simulink model "GalacticSoupLogical"  (R2026a)
settings: Solver=VariableStepAuto
settings Model: DataDictionary=LogicalInterfaces.sldd  Creator=sarah  LastModifiedBy=sarah

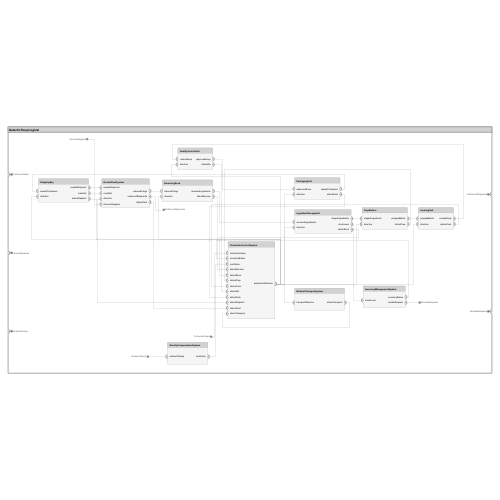
[thumbnail: Simulink's stored preview of the top-level diagram]
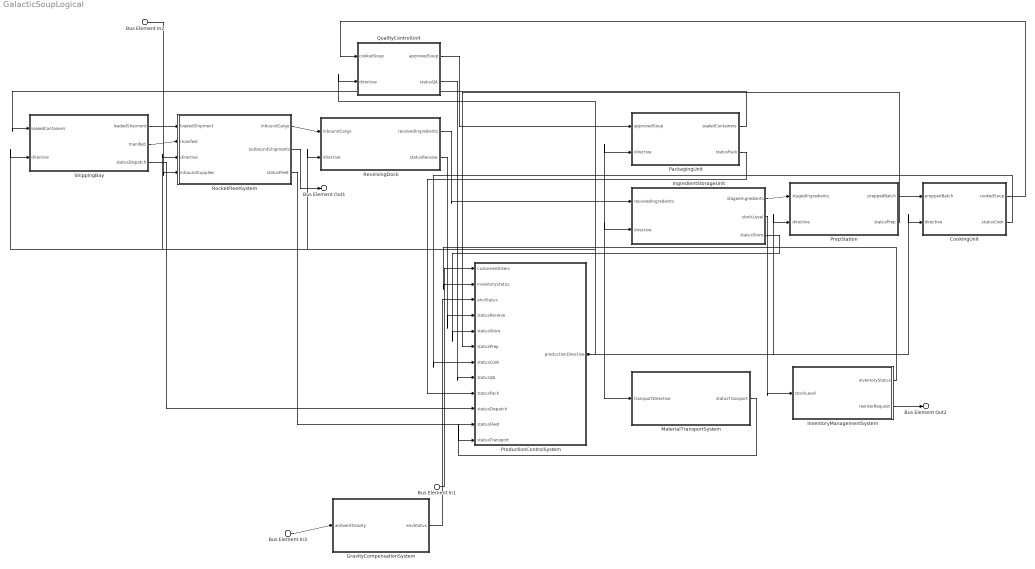
== system GalacticSoupLogical ==
  Bus Element In1 : Inport  PortName=CustomerOrders
  Bus Element In2 : Inport  Port=2  PortName=InboundSupplies
  Bus Element In3 : Inport  Port=3  PortName=AmbientGravity
  CookingUnit : Subsystem
      settings: PortSchema="{\"entries\":[{\"content\":{\"headerSize\":26,\"margin\":15,\"minimumSpacing\":25,\"sides\":[{\"content\":{\"connectorIds\":[\"In1\",\"In2\"]},\"type\":\"ConnectorPlacement.EquallySpacedRectSide\",\"uuid\":\"f830f98a-8e8b-4468-adf4-d6eab644987f\"},{\"content\":{\"connectorIds\":[\"Out1\",\"Out2\"],\"side\":\"RIGHT\"},\"type\":\"ConnectorPlacement.EquallySpacedRectSide\",\"uuid\":\"7e0d0116-b3ba-4668-b638-30d0f54ba087\"},{\"content\":{\"side\":\"TOP\"},\"type\":\"ConnectorPlacement.EquallySpacedRectSide\",\"uuid\":\"7b4146d3-46d2-45ca-8c34-b106f0d8cedd\"}]},\"type\":\"ConnectorPlacement.EquallySpacedConnector\",\"uuid\":\"3d911b2d-a78f-42ea-b869-5e09982d9f54\"}],\"packageUris\":[\"http://schema.mathworks.com/mf0/Connector/R2020b\"],\"version\":\"1.0\"}"
  GravityCompensationSystem : Subsystem
      settings: PortSchema="{\"entries\":[{\"content\":{\"headerSize\":26,\"margin\":15,\"minimumSpacing\":25,\"sides\":[{\"content\":{\"connectorIds\":[\"In1\"]},\"type\":\"ConnectorPlacement.EquallySpacedRectSide\",\"uuid\":\"f830f98a-8e8b-4468-adf4-d6eab644987f\"},{\"content\":{\"connectorIds\":[\"Out1\"],\"side\":\"RIGHT\"},\"type\":\"ConnectorPlacement.EquallySpacedRectSide\",\"uuid\":\"7e0d0116-b3ba-4668-b638-30d0f54ba087\"},{\"content\":{\"side\":\"TOP\"},\"type\":\"ConnectorPlacement.EquallySpacedRectSide\",\"uuid\":\"7b4146d3-46d2-45ca-8c34-b106f0d8cedd\"}]},\"type\":\"ConnectorPlacement.EquallySpacedConnector\",\"uuid\":\"3d911b2d-a78f-42ea-b869-5e09982d9f54\"}],\"packageUris\":[\"http://schema.mathworks.com/mf0/Connector/R2020b\"],\"version\":\"1.0\"}"
  IngredientStorageUnit : Subsystem
      settings: PortSchema="{\"entries\":[{\"content\":{\"headerSize\":26,\"margin\":15,\"minimumSpacing\":25,\"sides\":[{\"content\":{\"connectorIds\":[\"In1\",\"In2\"]},\"type\":\"ConnectorPlacement.EquallySpacedRectSide\",\"uuid\":\"f830f98a-8e8b-4468-adf4-d6eab644987f\"},{\"content\":{\"connectorIds\":[\"Out1\",\"Out2\",\"Out3\"],\"side\":\"RIGHT\"},\"type\":\"ConnectorPlacement.EquallySpacedRectSide\",\"uuid\":\"7e0d0116-b3ba-4668-b638-30d0f54ba087\"},{\"content\":{\"side\":\"TOP\"},\"type\":\"ConnectorPlacement.EquallySpacedRectSide\",\"uuid\":\"7b4146d3-46d2-45ca-8c34-b106f0d8cedd\"}]},\"type\":\"ConnectorPlacement.EquallySpacedConnector\",\"uuid\":\"3d911b2d-a78f-42ea-b869-5e09982d9f54\"}],\"packageUris\":[\"http://schema.mathworks.com/mf0/Connector/R2020b\"],\"version\":\"1.0\"}"
  InventoryManagementSystem : Subsystem
      settings: PortSchema="{\"entries\":[{\"content\":{\"headerSize\":26,\"margin\":15,\"minimumSpacing\":25,\"sides\":[{\"content\":{\"connectorIds\":[\"In1\"]},\"type\":\"ConnectorPlacement.EquallySpacedRectSide\",\"uuid\":\"f830f98a-8e8b-4468-adf4-d6eab644987f\"},{\"content\":{\"connectorIds\":[\"Out1\",\"Out2\"],\"side\":\"RIGHT\"},\"type\":\"ConnectorPlacement.EquallySpacedRectSide\",\"uuid\":\"7e0d0116-b3ba-4668-b638-30d0f54ba087\"},{\"content\":{\"side\":\"TOP\"},\"type\":\"ConnectorPlacement.EquallySpacedRectSide\",\"uuid\":\"7b4146d3-46d2-45ca-8c34-b106f0d8cedd\"}]},\"type\":\"ConnectorPlacement.EquallySpacedConnector\",\"uuid\":\"3d911b2d-a78f-42ea-b869-5e09982d9f54\"}],\"packageUris\":[\"http://schema.mathworks.com/mf0/Connector/R2020b\"],\"version\":\"1.0\"}"
  MaterialTransportSystem : Subsystem
      settings: PortSchema="{\"entries\":[{\"content\":{\"headerSize\":26,\"margin\":15,\"minimumSpacing\":25,\"sides\":[{\"content\":{\"connectorIds\":[\"In1\"]},\"type\":\"ConnectorPlacement.EquallySpacedRectSide\",\"uuid\":\"f830f98a-8e8b-4468-adf4-d6eab644987f\"},{\"content\":{\"connectorIds\":[\"Out1\"],\"side\":\"RIGHT\"},\"type\":\"ConnectorPlacement.EquallySpacedRectSide\",\"uuid\":\"7e0d0116-b3ba-4668-b638-30d0f54ba087\"},{\"content\":{\"side\":\"TOP\"},\"type\":\"ConnectorPlacement.EquallySpacedRectSide\",\"uuid\":\"7b4146d3-46d2-45ca-8c34-b106f0d8cedd\"}]},\"type\":\"ConnectorPlacement.EquallySpacedConnector\",\"uuid\":\"3d911b2d-a78f-42ea-b869-5e09982d9f54\"}],\"packageUris\":[\"http://schema.mathworks.com/mf0/Connector/R2020b\"],\"version\":\"1.0\"}"
  PackagingUnit : Subsystem
      settings: PortSchema="{\"entries\":[{\"content\":{\"headerSize\":26,\"margin\":15,\"minimumSpacing\":25,\"sides\":[{\"content\":{\"connectorIds\":[\"In1\",\"In2\"]},\"type\":\"ConnectorPlacement.EquallySpacedRectSide\",\"uuid\":\"f830f98a-8e8b-4468-adf4-d6eab644987f\"},{\"content\":{\"connectorIds\":[\"Out1\",\"Out2\"],\"side\":\"RIGHT\"},\"type\":\"ConnectorPlacement.EquallySpacedRectSide\",\"uuid\":\"7e0d0116-b3ba-4668-b638-30d0f54ba087\"},{\"content\":{\"side\":\"TOP\"},\"type\":\"ConnectorPlacement.EquallySpacedRectSide\",\"uuid\":\"7b4146d3-46d2-45ca-8c34-b106f0d8cedd\"}]},\"type\":\"ConnectorPlacement.EquallySpacedConnector\",\"uuid\":\"3d911b2d-a78f-42ea-b869-5e09982d9f54\"}],\"packageUris\":[\"http://schema.mathworks.com/mf0/Connector/R2020b\"],\"version\":\"1.0\"}"
  PrepStation : Subsystem
      settings: PortSchema="{\"entries\":[{\"content\":{\"headerSize\":26,\"margin\":15,\"minimumSpacing\":25,\"sides\":[{\"content\":{\"connectorIds\":[\"In1\",\"In2\"]},\"type\":\"ConnectorPlacement.EquallySpacedRectSide\",\"uuid\":\"f830f98a-8e8b-4468-adf4-d6eab644987f\"},{\"content\":{\"connectorIds\":[\"Out1\",\"Out2\"],\"side\":\"RIGHT\"},\"type\":\"ConnectorPlacement.EquallySpacedRectSide\",\"uuid\":\"7e0d0116-b3ba-4668-b638-30d0f54ba087\"},{\"content\":{\"side\":\"TOP\"},\"type\":\"ConnectorPlacement.EquallySpacedRectSide\",\"uuid\":\"7b4146d3-46d2-45ca-8c34-b106f0d8cedd\"}]},\"type\":\"ConnectorPlacement.EquallySpacedConnector\",\"uuid\":\"3d911b2d-a78f-42ea-b869-5e09982d9f54\"}],\"packageUris\":[\"http://schema.mathworks.com/mf0/Connector/R2020b\"],\"version\":\"1.0\"}"
  ProductionControlSystem : Subsystem
      settings: PortSchema="{\"entries\":[{\"content\":{\"headerSize\":26,\"margin\":15,\"minimumSpacing\":25,\"sides\":[{\"content\":{\"connectorIds\":[\"In1\",\"In2\",\"In3\",\"In4\",\"In5\",\"In6\",\"In7\",\"In8\",\"In9\",\"In10\",\"In11\",\"In12\"]},\"type\":\"ConnectorPlacement.EquallySpacedRectSide\",\"uuid\":\"f830f98a-8e8b-4468-adf4-d6eab644987f\"},{\"content\":{\"connectorIds\":[\"Out1\"],\"side\":\"RIGHT\"},\"type\":\"ConnectorPlacement.EquallySpacedRectSide\",\"uuid\":\"7e0d0116-b3ba-4668-b638-30d0f54ba087\"},{\"content\":{\"side\":\"TOP\"},\"type\":\"ConnectorPlacement.EquallySpacedRectSide\",\"uuid\":\"7b4146d3-46d2-45ca-8c34-b106f0d8cedd\"}]},\"type\":\"ConnectorPlacement.EquallySpacedConnector\",\"uuid\":\"3d911b2d-a78f-42ea-b869-5e09982d9f54\"}],\"packageUris\":[\"http://schema.mathworks.com/mf0/Connector/R2020b\"],\"version\":\"1.0\"}"
  QualityControlUnit : Subsystem
      settings: PortSchema="{\"entries\":[{\"content\":{\"headerSize\":26,\"margin\":15,\"minimumSpacing\":25,\"sides\":[{\"content\":{\"connectorIds\":[\"In1\",\"In2\"]},\"type\":\"ConnectorPlacement.EquallySpacedRectSide\",\"uuid\":\"f830f98a-8e8b-4468-adf4-d6eab644987f\"},{\"content\":{\"connectorIds\":[\"Out1\",\"Out2\"],\"side\":\"RIGHT\"},\"type\":\"ConnectorPlacement.EquallySpacedRectSide\",\"uuid\":\"7e0d0116-b3ba-4668-b638-30d0f54ba087\"},{\"content\":{\"side\":\"TOP\"},\"type\":\"ConnectorPlacement.EquallySpacedRectSide\",\"uuid\":\"7b4146d3-46d2-45ca-8c34-b106f0d8cedd\"}]},\"type\":\"ConnectorPlacement.EquallySpacedConnector\",\"uuid\":\"3d911b2d-a78f-42ea-b869-5e09982d9f54\"}],\"packageUris\":[\"http://schema.mathworks.com/mf0/Connector/R2020b\"],\"version\":\"1.0\"}"
  ReceivingDock : Subsystem
      settings: PortSchema="{\"entries\":[{\"content\":{\"headerSize\":26,\"margin\":15,\"minimumSpacing\":25,\"sides\":[{\"content\":{\"connectorIds\":[\"In1\",\"In2\"]},\"type\":\"ConnectorPlacement.EquallySpacedRectSide\",\"uuid\":\"f830f98a-8e8b-4468-adf4-d6eab644987f\"},{\"content\":{\"connectorIds\":[\"Out1\",\"Out2\"],\"side\":\"RIGHT\"},\"type\":\"ConnectorPlacement.EquallySpacedRectSide\",\"uuid\":\"7e0d0116-b3ba-4668-b638-30d0f54ba087\"},{\"content\":{\"side\":\"TOP\"},\"type\":\"ConnectorPlacement.EquallySpacedRectSide\",\"uuid\":\"7b4146d3-46d2-45ca-8c34-b106f0d8cedd\"}]},\"type\":\"ConnectorPlacement.EquallySpacedConnector\",\"uuid\":\"3d911b2d-a78f-42ea-b869-5e09982d9f54\"}],\"packageUris\":[\"http://schema.mathworks.com/mf0/Connector/R2020b\"],\"version\":\"1.0\"}"
  RocketFleetSystem : Subsystem
      settings: PortSchema="{\"entries\":[{\"content\":{\"headerSize\":26,\"margin\":15,\"minimumSpacing\":25,\"sides\":[{\"content\":{\"connectorIds\":[\"In1\",\"In2\",\"In3\",\"In4\"]},\"type\":\"ConnectorPlacement.EquallySpacedRectSide\",\"uuid\":\"f830f98a-8e8b-4468-adf4-d6eab644987f\"},{\"content\":{\"connectorIds\":[\"Out1\",\"Out2\",\"Out3\"],\"side\":\"RIGHT\"},\"type\":\"ConnectorPlacement.EquallySpacedRectSide\",\"uuid\":\"7e0d0116-b3ba-4668-b638-30d0f54ba087\"},{\"content\":{\"side\":\"TOP\"},\"type\":\"ConnectorPlacement.EquallySpacedRectSide\",\"uuid\":\"7b4146d3-46d2-45ca-8c34-b106f0d8cedd\"}]},\"type\":\"ConnectorPlacement.EquallySpacedConnector\",\"uuid\":\"3d911b2d-a78f-42ea-b869-5e09982d9f54\"}],\"packageUris\":[\"http://schema.mathworks.com/mf0/Connector/R2020b\"],\"version\":\"1.0\"}"
  ShippingBay : Subsystem
      settings: PortSchema="{\"entries\":[{\"content\":{\"headerSize\":26,\"margin\":15,\"minimumSpacing\":25,\"sides\":[{\"content\":{\"connectorIds\":[\"In1\",\"In2\"]},\"type\":\"ConnectorPlacement.EquallySpacedRectSide\",\"uuid\":\"f830f98a-8e8b-4468-adf4-d6eab644987f\"},{\"content\":{\"connectorIds\":[\"Out1\",\"Out2\",\"Out3\"],\"side\":\"RIGHT\"},\"type\":\"ConnectorPlacement.EquallySpacedRectSide\",\"uuid\":\"7e0d0116-b3ba-4668-b638-30d0f54ba087\"},{\"content\":{\"side\":\"TOP\"},\"type\":\"ConnectorPlacement.EquallySpacedRectSide\",\"uuid\":\"7b4146d3-46d2-45ca-8c34-b106f0d8cedd\"}]},\"type\":\"ConnectorPlacement.EquallySpacedConnector\",\"uuid\":\"3d911b2d-a78f-42ea-b869-5e09982d9f54\"}],\"packageUris\":[\"http://schema.mathworks.com/mf0/Connector/R2020b\"],\"version\":\"1.0\"}"
  Bus Element Out1 : Outport  PortName=OutboundShipments
  Bus Element Out2 : Outport  Port=2  PortName=ReorderRequests
  wires:
  Bus Element In2/1 -> RocketFleetSystem/4(inboundSupplies)
  RocketFleetSystem/1(inboundCargo) -> ReceivingDock/1(inboundCargo)
  ShippingBay/3(statusDispatch) -> ProductionControlSystem/10(statusDispatch)
  Bus Element In3/1 -> GravityCompensationSystem/1(ambientGravity)
  ShippingBay/1(loadedShipment) -> RocketFleetSystem/1(loadedShipment)
  ShippingBay/2(manifest) -> RocketFleetSystem/2(manifest)
  CookingUnit/1(cookedSoup) -> QualityControlUnit/1(cookedSoup)
  RocketFleetSystem/2(outboundShipments) -> Bus Element Out1/1
  CookingUnit/2(statusCook) -> ProductionControlSystem/7(statusCook)
  RocketFleetSystem/3(statusFleet) -> ProductionControlSystem/11(statusFleet)
  QualityControlUnit/1(approvedSoup) -> PackagingUnit/1(approvedSoup)
  QualityControlUnit/2(statusQA) -> ProductionControlSystem/8(statusQA)
  ReceivingDock/1(receivedIngredients) -> IngredientStorageUnit/1(receivedIngredients)
  ReceivingDock/2(statusReceive) -> ProductionControlSystem/4(statusReceive)
  Bus Element In1/1 -> ProductionControlSystem/1(customerOrders)
  GravityCompensationSystem/1(envStatus) -> ProductionControlSystem/3(envStatus)
  ProductionControlSystem/1(productionDirective) -> ReceivingDock/2(directive), ShippingBay/2(directive), QualityControlUnit/2(directive), RocketFleetSystem/3(directive), PrepStation/2(directive), CookingUnit/2(directive), IngredientStorageUnit/2(directive), PackagingUnit/2(directive), MaterialTransportSystem/1(transportDirective)
  PackagingUnit/1(sealedContainers) -> ShippingBay/1(sealedContainers)
  PackagingUnit/2(statusPack) -> ProductionControlSystem/9(statusPack)
  IngredientStorageUnit/1(stagedIngredients) -> PrepStation/1(stagedIngredients)
  IngredientStorageUnit/2(stockLevel) -> InventoryManagementSystem/1(stockLevel)
  IngredientStorageUnit/3(statusStore) -> ProductionControlSystem/5(statusStore)
  MaterialTransportSystem/1(statusTransport) -> ProductionControlSystem/12(statusTransport)
  PrepStation/1(preppedBatch) -> CookingUnit/1(preppedBatch)
  PrepStation/2(statusPrep) -> ProductionControlSystem/6(statusPrep)
  InventoryManagementSystem/1(inventoryStatus) -> ProductionControlSystem/2(inventoryStatus)
  InventoryManagementSystem/2(reorderRequest) -> Bus Element Out2/1

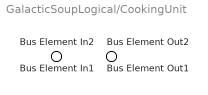
== system GalacticSoupLogical/CookingUnit ==
  Bus Element In1 : Inport  PortName=preppedBatch
  Bus Element In2 : Inport  Port=2  PortName=directive
  Bus Element Out1 : Outport  PortName=cookedSoup
  Bus Element Out2 : Outport  Port=2  PortName=statusCook

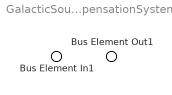
== system GalacticSoupLogical/GravityCompensationSystem ==
  Bus Element In1 : Inport  PortName=ambientGravity
  Bus Element Out1 : Outport  PortName=envStatus

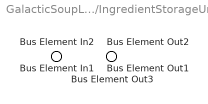
== system GalacticSoupLogical/IngredientStorageUnit ==
  Bus Element In1 : Inport  PortName=receivedIngredients
  Bus Element In2 : Inport  Port=2  PortName=directive
  Bus Element Out1 : Outport  PortName=stagedIngredients
  Bus Element Out2 : Outport  Port=2  PortName=stockLevel
  Bus Element Out3 : Outport  Port=3  PortName=statusStore

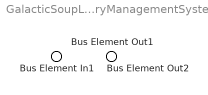
== system GalacticSoupLogical/InventoryManagementSystem ==
  Bus Element In1 : Inport  PortName=stockLevel
  Bus Element Out1 : Outport  PortName=inventoryStatus
  Bus Element Out2 : Outport  Port=2  PortName=reorderRequest

== system GalacticSoupLogical/MaterialTransportSystem ==
  Bus Element In1 : Inport  PortName=transportDirective
  Bus Element Out1 : Outport  PortName=statusTransport

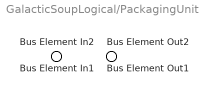
== system GalacticSoupLogical/PackagingUnit ==
  Bus Element In1 : Inport  PortName=approvedSoup
  Bus Element In2 : Inport  Port=2  PortName=directive
  Bus Element Out1 : Outport  PortName=sealedContainers
  Bus Element Out2 : Outport  Port=2  PortName=statusPack

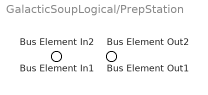
== system GalacticSoupLogical/PrepStation ==
  Bus Element In1 : Inport  PortName=stagedIngredients
  Bus Element In2 : Inport  Port=2  PortName=directive
  Bus Element Out1 : Outport  PortName=preppedBatch
  Bus Element Out2 : Outport  Port=2  PortName=statusPrep

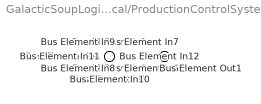
== system GalacticSoupLogical/ProductionControlSystem ==
  Bus Element In1 : Inport  PortName=customerOrders
  Bus Element In2 : Inport  Port=2  PortName=inventoryStatus
  Bus Element In3 : Inport  Port=3  PortName=envStatus
  Bus Element In4 : Inport  Port=4  PortName=statusReceive
  Bus Element In5 : Inport  Port=5  PortName=statusStore
  Bus Element In6 : Inport  Port=6  PortName=statusPrep
  Bus Element In7 : Inport  Port=7  PortName=statusCook
  Bus Element In8 : Inport  Port=8  PortName=statusQA
  Bus Element In9 : Inport  Port=9  PortName=statusPack
  Bus Element In10 : Inport  Port=10  PortName=statusDispatch
  Bus Element In11 : Inport  Port=11  PortName=statusFleet
  Bus Element In12 : Inport  Port=12  PortName=statusTransport
  Bus Element Out1 : Outport  PortName=productionDirective

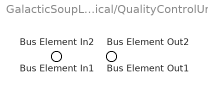
== system GalacticSoupLogical/QualityControlUnit ==
  Bus Element In1 : Inport  PortName=cookedSoup
  Bus Element In2 : Inport  Port=2  PortName=directive
  Bus Element Out1 : Outport  PortName=approvedSoup
  Bus Element Out2 : Outport  Port=2  PortName=statusQA

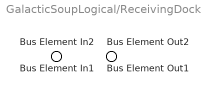
== system GalacticSoupLogical/ReceivingDock ==
  Bus Element In1 : Inport  PortName=inboundCargo
  Bus Element In2 : Inport  Port=2  PortName=directive
  Bus Element Out1 : Outport  PortName=receivedIngredients
  Bus Element Out2 : Outport  Port=2  PortName=statusReceive

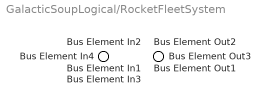
== system GalacticSoupLogical/RocketFleetSystem ==
  Bus Element In1 : Inport  PortName=loadedShipment
  Bus Element In2 : Inport  Port=2  PortName=manifest
  Bus Element In3 : Inport  Port=3  PortName=directive
  Bus Element In4 : Inport  Port=4  PortName=inboundSupplies
  Bus Element Out1 : Outport  PortName=inboundCargo
  Bus Element Out2 : Outport  Port=2  PortName=outboundShipments
  Bus Element Out3 : Outport  Port=3  PortName=statusFleet

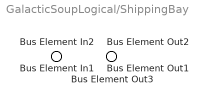
== system GalacticSoupLogical/ShippingBay ==
  Bus Element In1 : Inport  PortName=sealedContainers
  Bus Element In2 : Inport  Port=2  PortName=directive
  Bus Element Out1 : Outport  PortName=loadedShipment
  Bus Element Out2 : Outport  Port=2  PortName=manifest
  Bus Element Out3 : Outport  Port=3  PortName=statusDispatch
